simulink model "untitled1"  (R2022a)
settings: Solver=ode23t  StartTime=0.0  StopTime=2  RelTol=1e-3
libraries: spsSeriesRLCBranchLib x23, spsIdealSwitchLib x22, spsDiodeLib x10, spsPVArrayLib x9, spsVoltageMeasurementLib x2, spsMosfetLib x1, spsCurrentMeasurementLib x1, spspowerguiLib x1
settings Model: Creator=Dell  LastModifiedBy=Dell

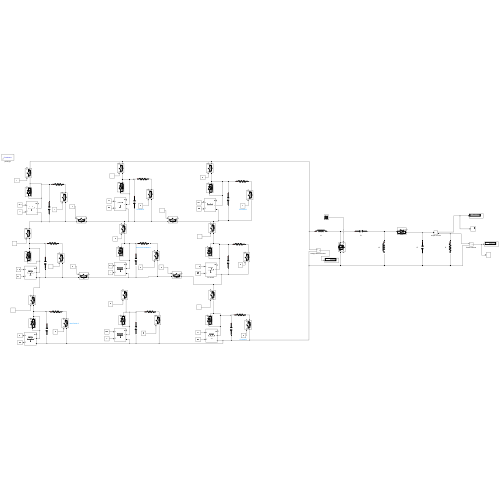
[thumbnail: Simulink's stored preview of the top-level diagram]
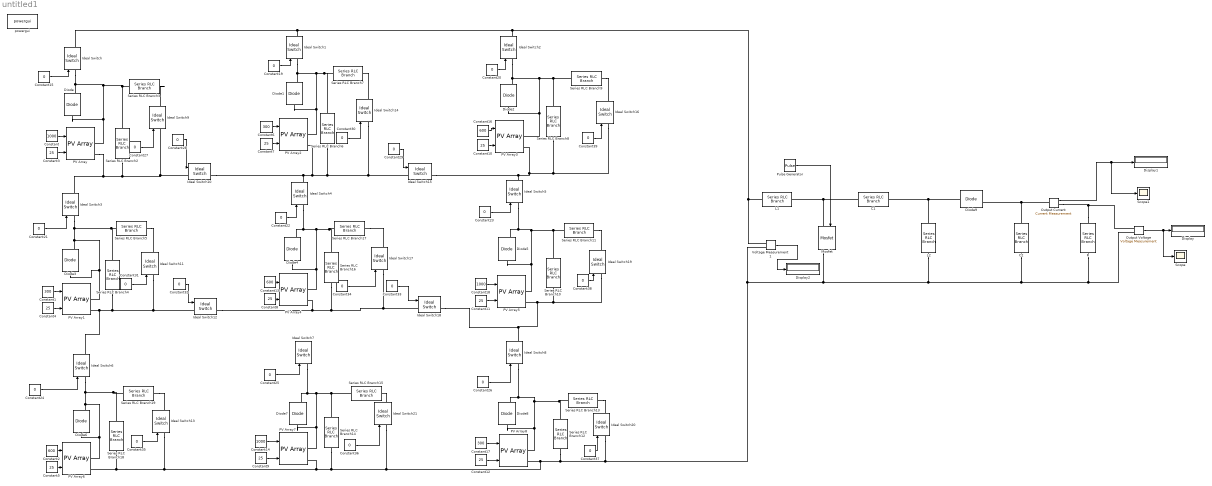
== system untitled1 ==
  C1 : spsSeriesRLCBranchLib/Series RLC Branch  LConnTagsString=__new0  RConnTagsString=__new0  BranchType=C  Resistance=1  Inductance=1e-3  SetiL0=off  InitialCurrent=0  Capacitance=28.57e-6  Setx0=off  InitialVoltage=0  Measurements=None
  C2 : spsSeriesRLCBranchLib/Series RLC Branch  LConnTagsString=__new0  RConnTagsString=__new0  BranchType=C  Resistance=1  Inductance=1e-3  SetiL0=off  InitialCurrent=0  Capacitance=28.57e-6  Setx0=off  InitialVoltage=0  Measurements=None
  Constant : Constant  Value=1000
  Constant1 : Constant  Value=300
  Constant{3..5,7..12} (9 alike) : Constant  Value=25
  Constant13 : Constant  Value=600
  Constant14 : Constant  Value=1000
  Constant{15,19..39} (22 alike) : Constant  Value=0
  Constant16 : Constant  Value=600
  Constant17 : Constant  Value=300
  Constant18 : Constant  Value=1000
  Constant2 : Constant  Value=600
  Constant6 : Constant  Value=300
  Diode{,1..9} (10 alike) : spsDiodeLib/Diode  Ron=0.001  Lon=0  Vf=0.8  IC=0  UseSnubber=0  Rs=500  Cs=250e-9  Measurements=on
  Display : Display
  Display1 : Display
  Display2 : Display
  Ideal Switch{,1..21} (22 alike) : spsIdealSwitchLib/Ideal Switch  Ron=0.001  Lon=0  IC=0  Rs=1e5  Cs=inf  Measurements=on
  L1 : spsSeriesRLCBranchLib/Series RLC Branch  LConnTagsString=__new0  RConnTagsString=__new0  BranchType=L  Resistance=1  Inductance=35.62e-6  SetiL0=off  InitialCurrent=0  Capacitance=1e-6  Setx0=off  InitialVoltage=0  Measurements=None
  L2 : spsSeriesRLCBranchLib/Series RLC Branch  LConnTagsString=__new0  RConnTagsString=__new0  BranchType=L  Resistance=1  Inductance=14.25e-6  SetiL0=off  InitialCurrent=0  Capacitance=1e-6  Setx0=off  InitialVoltage=0  Measurements=None
  Mosfet : spsMosfetLib/Mosfet  Ron=0.1  Lon=0  Rd=0.01  Vfd=0  IC=0  Rs=1e5  Cs=inf  Measurements=on
  Output Current : spsCurrentMeasurementLib/Current Measurement  PhasorSimulation=off  OutputType=Complex  PSBequivalent=0
  Output Voltage : spsVoltageMeasurementLib/Voltage Measurement  PhasorSimulation=off  OutputType=Complex  PSBequivalent=0
  PV Array{,1..8} (9 alike) : spsPVArrayLib/PV Array  Npar=1  Nser=1  PlotType=array @ 1000 W/m2 & specified temperatures  S_vec="[ 1000  500  100 ]"  Temp_C_vec="[ 45 25  ]"  ModuleName=Aavid Solar ASMS-165P  PlotWhenSelected=off  Pm=164.85  Ncell=72  Voc=43.5  Isc=5.25  Vm=35  Im=4.71  beta_Voc_pc=-0.393  alpha_Isc_pc=0.03  beta_Voc=-0.17095  alpha_Isc=0.001575  IL=5.2764  I0=4.9875e-10  nI=1.0218  Rsh=125.0069  Rs=0.62818  RobustModel=off  RobustCellTemperature=313.3991  BAL=on  Tc=1e-6  Tfilter=5e-5
  Pulse Generator : DiscretePulseGenerator  PulseType=Time based  Period=1/250e3  PulseWidth=28.57
  R : spsSeriesRLCBranchLib/Series RLC Branch  LConnTagsString=__new0  RConnTagsString=__new0  BranchType=R  Resistance=20  Inductance=1e-3  SetiL0=off  InitialCurrent=0  Capacitance=1e-6  Setx0=off  InitialVoltage=0  Measurements=None
  Scope : Scope
  Scope1 : Scope
  Series RLC Branch{2,4,6,8,10,12,14,16,18} (9 alike) : spsSeriesRLCBranchLib/Series RLC Branch  LConnTagsString=__new0  RConnTagsString=__new0  BranchType=C  Resistance=1  Inductance=1e-3  SetiL0=off  InitialCurrent=0  Capacitance=1e-6  Setx0=off  InitialVoltage=0  Measurements=None
  Series RLC Branch{3,5,7,9,11,13,15,17,19} (9 alike) : spsSeriesRLCBranchLib/Series RLC Branch  LConnTagsString=__new0  RConnTagsString=__new0  BranchType=R  Resistance=1  Inductance=1e-3  SetiL0=off  InitialCurrent=0  Capacitance=1e-6  Setx0=off  InitialVoltage=0  Measurements=None
  "Voltage Measurement1 " : spsVoltageMeasurementLib/Voltage Measurement  PhasorSimulation=off  OutputType=Complex  PSBequivalent=0
  powergui : spspowerguiLib/powergui  Priority=1  SimulationMode=Continuous  SampleTime=1  frequency=60  Iterations=50  frequencyindice=0  Pbase=100e6  ErrMax=1e-4  UnitsV=kV  UnitsW=MW  buscounter=0  FunctionMessages=off  echomessages=off  EnableUseOfTLC=off  CurrentSourceSwitches=off  DisableSnubberDevices=off  DisableRonSwitches=off  DisableVfSwitches=off  DisplayEquations=off  AutomaticDiscreteSolvers=off  SolverType=Tustin/Backward Euler (TBE)  Interpol=off  ExternalGateDelay=off  methode=off  Ts=100  x0status=blocks  SPID=on  SwTol=0  HookPort=off  NonlinearTolerance=1e-4  nMaxIteration=100  ContinueOnMaxIteration=off  RestoreLinks=warning  ResistiveCurrentMeasurement=off  Frange=[0:2:500]  Ylog=off  Xlog=on  ShowGrid=off  save=off  variable=ZData  structure=0  ZoomFFT=off  StartTime=0.0  cycles=1  DisplayStyle=1  fundamental=60  FreqAxis=off  MaxFrequency=1000  frequencyindicesteady=1  RmsSteady=1  display=off
  wires:
  Constant/1 -> PV Array/1
  Constant2/1 -> PV Array6/1
  Constant1/1 -> PV Array1/1
  Constant3/1 -> PV Array/2
  Constant4/1 -> PV Array1/2
  Constant5/1 -> PV Array6/2
  Constant6/1 -> PV Array2/1
  Constant12/1 -> PV Array8/2
  Constant11/1 -> PV Array5/2
  Constant10/1 -> PV Array3/2
  Constant7/1 -> PV Array2/2
  Constant8/1 -> PV Array4/2
  Constant9/1 -> PV Array7/2
  Constant13/1 -> PV Array4/1
  Constant14/1 -> PV Array7/1
  Constant16/1 -> PV Array3/1
  Constant18/1 -> PV Array5/1
  Constant17/1 -> PV Array8/1
  Constant15/1 -> Ideal Switch/1
  Constant19/1 -> Ideal Switch1/1
  Constant20/1 -> Ideal Switch2/1
  Constant21/1 -> Ideal Switch3/1
  Constant22/1 -> Ideal Switch4/1
  Constant23/1 -> Ideal Switch5/1
  Constant24/1 -> Ideal Switch6/1
  Constant25/1 -> Ideal Switch7/1
  Constant26/1 -> Ideal Switch8/1
  Constant27/1 -> Ideal Switch9/1
  Constant28/1 -> Ideal Switch10/1
  Constant30/1 -> Ideal Switch14/1
  Constant29/1 -> Ideal Switch15/1
  Constant39/1 -> Ideal Switch16/1
  Constant38/1 -> Ideal Switch19/1
  Constant37/1 -> Ideal Switch20/1
  Constant36/1 -> Ideal Switch21/1
  Constant34/1 -> Ideal Switch17/1
  Constant33/1 -> Ideal Switch18/1
  Constant32/1 -> Ideal Switch12/1
  Constant31/1 -> Ideal Switch11/1
  Constant35/1 -> Ideal Switch13/1
  Output Voltage/1 -> Scope/1, Display/1
  Pulse Generator/1 -> Mosfet/1
  Output Current/1 -> Scope1/1, Display1/1
  "Voltage Measurement1 "/1 -> Display2/1
  connections:
  Diode/RConn1 -- Ideal Switch/LConn1 -- Series RLC Branch2/LConn1 -- Series RLC Branch3/LConn1 -- Diode/LConn1 -- PV Array/RConn1
  Diode1/RConn1 -- Ideal Switch1/LConn1 -- Series RLC Branch7/LConn1 -- Series RLC Branch6/LConn1 -- Diode1/LConn1 -- PV Array2/RConn1
  Diode2/RConn1 -- Ideal Switch2/LConn1 -- Series RLC Branch9/LConn1 -- Series RLC Branch8/LConn1 -- Diode2/LConn1 -- PV Array3/RConn1
  Diode3/RConn1 -- Series RLC Branch4/LConn1 -- Series RLC Branch5/LConn1 -- Ideal Switch3/LConn1 -- Diode3/LConn1 -- PV Array1/RConn1
  Diode4/RConn1 -- Ideal Switch4/LConn1 -- Series RLC Branch17/LConn1 -- Series RLC Branch16/LConn1 -- Diode4/LConn1 -- PV Array4/RConn1
  Diode5/RConn1 -- Ideal Switch5/LConn1 -- Series RLC Branch11/LConn1 -- Series RLC Branch10/LConn1 -- Diode5/LConn1 -- PV Array5/RConn1
  Diode6/RConn1 -- Series RLC Branch19/LConn1 -- Series RLC Branch18/LConn1 -- Ideal Switch6/LConn1 -- Diode6/LConn1 -- PV Array6/RConn1
  Diode7/RConn1 -- Ideal Switch7/LConn1 -- Series RLC Branch15/LConn1 -- Series RLC Branch14/LConn1 -- Diode7/LConn1 -- PV Array7/RConn1
  Diode8/RConn1 -- Ideal Switch8/LConn1 -- Series RLC Branch13/LConn1 -- Series RLC Branch12/LConn1 -- Diode8/LConn1 -- PV Array8/RConn1
  PV Array/RConn2 -- Ideal Switch3/RConn1 -- Series RLC Branch2/RConn1 -- Ideal Switch10/LConn1 -- Ideal Switch9/LConn1
  Ideal Switch10/RConn1 -- Ideal Switch4/RConn1 -- Ideal Switch14/LConn1 -- Ideal Switch15/LConn1 -- Series RLC Branch6/RConn1 -- PV Array2/RConn2
  Ideal Switch11/LConn1 -- Series RLC Branch4/RConn1 -- Ideal Switch6/RConn1 -- PV Array1/RConn2 -- Ideal Switch12/LConn1
  Ideal Switch12/RConn1 -- Ideal Switch18/LConn1 -- Ideal Switch17/LConn1 -- Series RLC Branch16/RConn1 -- PV Array4/RConn2
  Ideal Switch15/RConn1 -- Ideal Switch5/RConn1 -- Series RLC Branch8/RConn1 -- Ideal Switch16/LConn1 -- PV Array3/RConn2
  L2/RConn1 -- Mosfet/RConn1 -- Series RLC Branch12/RConn1 -- Series RLC Branch14/RConn1 -- Series RLC Branch18/RConn1 -- PV Array6/RConn2 -- Ideal Switch13/LConn1 -- PV Array7/RConn2 -- Ideal Switch21/LConn1 -- PV Array8/RConn2 -- Ideal Switch20/LConn1 -- "Voltage Measurement1 "/LConn2 -- Output Voltage/LConn2 -- R/RConn1 -- C2/RConn1
  Ideal Switch19/LConn1 -- Series RLC Branch10/RConn1 -- Ideal Switch8/RConn1 -- Ideal Switch18/RConn1 -- PV Array5/RConn2
  L1/LConn1 -- Ideal Switch/RConn1 -- Ideal Switch1/RConn1 -- Ideal Switch2/RConn1 -- "Voltage Measurement1 "/LConn1
  Diode9/RConn1 -- C2/LConn1 -- Output Current/LConn1
  R/LConn1 -- Output Current/RConn1 -- Output Voltage/LConn1
  C1/LConn1 -- Mosfet/LConn1 -- L1/RConn1
  C1/RConn1 -- L2/LConn1 -- Diode9/LConn1
  Series RLC Branch3/RConn1 -- Ideal Switch9/RConn1
  Series RLC Branch5/RConn1 -- Ideal Switch11/RConn1
  Series RLC Branch7/RConn1 -- Ideal Switch14/RConn1
  Series RLC Branch9/RConn1 -- Ideal Switch16/RConn1
  Series RLC Branch11/RConn1 -- Ideal Switch19/RConn1
  Series RLC Branch13/RConn1 -- Ideal Switch20/RConn1
  Series RLC Branch15/RConn1 -- Ideal Switch21/RConn1
  Series RLC Branch17/RConn1 -- Ideal Switch17/RConn1
  Series RLC Branch19/RConn1 -- Ideal Switch13/RConn1
